simulink model "hpt_v2_topology2_paper"  (R2025a)
settings: Solver=ode23tb  StartTime=0.0  StopTime=0.2  RelTol=1e-3
model workspace (MAT data in the model file):
  hpt_chopper_threshold = 850
  hpt_conventional_energy_scale = 1
  hpt_conventional_energy_scale_sag = 1
  hpt_conventional_energy_scale_swell = 1
  hpt_conventional_recovery_hold_s = 0
  hpt_conventional_recovery_reg_gain = 0
  hpt_conventional_recovery_reg_max = 0
  hpt_conventional_reg_scale = 1
  hpt_conventional_reg_scale_sag = 1
  hpt_conventional_reg_scale_swell = 1
  hpt_ctrl_Ts = 2e-05
  hpt_energy_bridge_polarity = -1
  hpt_energy_control_sign = -1
  hpt_energy_i_ki = 100
  hpt_energy_i_kp = 0.5
  hpt_energy_id_max = 20
  hpt_energy_vff_gain = 1.06
  hpt_grid_f0 = 50
  hpt_inj_phase_offset = -1.05
  hpt_m_energy = 0
  hpt_m_energy_max = 0.95
  hpt_m_reg = 0.1
  hpt_m_reg_max = 0.8
  hpt_pll_ki = 2500
  hpt_pll_kp = 80
  hpt_pwm_fs = 2000
  hpt_rchop = 5.33333333333
  hpt_reg_openloop_amp = 0
  hpt_reg_openloop_phase = 0
  hpt_reg_polarity = 1
  hpt_s2_resistance = 0.001
  hpt_sac_actor_filter_tau = 0.001
  hpt_sac_actor_select_mode = 0
  hpt_sac_dynamic_reg_limit = 0.6
  hpt_sac_enable = 0
  hpt_sac_energy_enable = 0
  hpt_sac_energy_max = 0.95
  hpt_sac_fault_time_norm_s = 0.5
  hpt_sac_fixed_energy_d = 0
  hpt_sac_fixed_energy_q = 0
  hpt_sac_fixed_reg_d = 0
  hpt_sac_fixed_reg_q = 0
  hpt_sac_grid_vref_phase = 5773.5026919
  hpt_sac_gridnorm_startup_s = 0.03
  hpt_sac_guard_enable = 0
  hpt_sac_i_base_peak = 816.496580928
  hpt_sac_phase_fault_clear_s = 0
  hpt_sac_phase_fault_start_s = 0
  hpt_sac_phase_override_enable = 0
  hpt_sac_phase_recovery_end_s = 0
  hpt_sac_policy_mode = 0
  hpt_sac_recovery_time_norm_s = 0.5
  hpt_sac_reg_d_gain = 1
  hpt_sac_reg_max = 0.8
  hpt_sac_reg_polarity = 1
  hpt_sac_reg_q_gain = 1
  hpt_sac_topology_id = 2
  hpt_sac_vdc_ref = 800
  hpt_sac_vref_phase = 230
  hpt_swell_gain_scale = 1
  hpt_swell_m_reg_max = 0.5
  hpt_swell_phase_offset = -0.5
  hpt_traj_action = [0  0  0  0; 0  0  0  0; 0  0  0  0; 0  0  0  0; 0  0  0  0; 0  0  0  0; 0  0  0  0; 0  0  0  0; 0  0  0  0; 0  0  0  0; 0  0  0  0; 0  0  0  0; 0  0  0  0; 0  0  0  0; 0  0  0  0; 0  0  0  0; 0  0  0  0; 0  0  0  0; 0  0  0  0; 0  0  0  0; 0  0  0  0; 0  0  0  0; 0  0  0  0; 0  0  0  0; 0  0  0  0; 0  0  0  0; 0  0  0  0; 0  0  0  0; 0  0  0  0; 0  0  0  0; 0  0  0  0; 0  0  0  0; 0  0  0  0; 0  0  0  0; 0  0  0  0; 0  0  0  0; 0  0  0  0; 0  0  0  0; 0  0  0  0; 0  0  0  0; 0  0  0  0; 0  0  0  0; 0  0  0  0; 0  0  0  0; 0  0  0  0; 0  0  0  0; 0  0  0  0; 0  0  0  0; 0  0  0  0; 0  0  0  0; 0  0  0  0; 0  0  0  0; 0  0  0  0; 0  0  0  0; 0  0  0  0; 0  0  0  0; 0  0  0  0; 0  0  0  0; 0  0  0  0; 0  0  0  0; 0  0  0  0; 0  0  0  0; 0  0  0  0; 0  0  0  0; 0  0  0  0; 0  0  0  0; 0  0  0  0; 0  0  0  0; 0  0  0  0; 0  0  0  0; 0  0  0  0; 0  0  0  0; 0  0  0  0; 0  0  0  0; 0  0  0  0; 0  0  0  0; 0  0  0  0; 0  0  0  0; 0  0  0  0; 0  0  0  0; 0  0  0  0; 0  0  0  0; 0  0  0  0; 0  0  0  0; 0  0  0  0; 0  0  0  0; 0  0  0  0; 0  0  0  0; 0  0  0  0; 0  0  0  0; 0  0  0  0; 0  0  0  0; 0  0  0  0; 0  0  0  0; 0  0  0  0; 0  0  0  0; 0  0  0  0; 0  0  0  0; 0  0  0  0; 0  0  0  0; 0  0  0  0; 0  0  0  0; 0  0  0  0; 0  0  0  0; 0  0  0  0; 0  0  0  0; 0  0  0  0; 0  0  0  0; 0  0  0  0; 0  0  0  0; 0  0  0  0; 0  0  0  0; 0  0  0  0; 0  0  0  0; 0  0  0  0; 0  0  0  0; 0  0  0  0; 0  0  0  0; 0  0  0  0; 0  0  0  0; 0  0  0  0; 0  0  0  0; 0  0  0  0; 0  0  0  0; 0  0  0  0; 0  0  0  0]
  hpt_traj_t = [0; 0.002; 0.004; 0.006; 0.008; 0.01; 0.012; 0.014; 0.016; 0.018; 0.02; 0.022; 0.024; 0.026; 0.028; 0.03; 0.032; 0.034; 0.036; 0.038; 0.04; 0.042; 0.044; 0.046; 0.048; 0.05; 0.052; 0.054; 0.056; 0.058; 0.06; 0.062; 0.064; 0.066; 0.068; 0.07; 0.072; 0.074; 0.076; 0.078; 0.08; 0.082; 0.084; 0.086; 0.088; 0.09; 0.092; 0.094; 0.096; 0.098; 0.1; 0.102; 0.104; 0.106; 0.108; 0.11; 0.112; 0.114; 0.116; 0.118; 0.12; 0.122; 0.124; 0.126; 0.128; 0.13; 0.132; 0.134; 0.136; 0.138; 0.14; 0.142; 0.144; 0.146; 0.148; 0.15; 0.152; 0.154; 0.156; 0.158; 0.16; 0.162; 0.164; 0.166; 0.168; 0.17; 0.172; 0.174; 0.176; 0.178; 0.18; 0.182; 0.184; 0.186; 0.188; 0.19; 0.192; 0.194; 0.196; 0.198; 0.2; 0.202; 0.204; 0.206; 0.208; 0.21; 0.212; 0.214; 0.216; 0.218; 0.22; 0.222; 0.224; 0.226; 0.228; 0.23; 0.232; 0.234; 0.236; 0.238; 0.24; 0.242; 0.244; 0.246; 0.248; 0.25]
  hpt_vdc_ki = 0.2
  hpt_vdc_kp = 2
  hpt_vdc_ref = 800
  hpt_vref_lv = 207
  hpt_vreg_ki = 0
  hpt_vreg_kp = 20
libraries: spsSeriesRLCBranchLib x17, spsVoltageMeasurementLib x10, spsLinearTransformerLib x9, simulink x9, spsGroundLib x5, spsUniversalBridgeLib x4, spsThreePhaseVIMeasurementLib x3, spsCurrentMeasurementLib x3, spsIGBTLib x1, spsThreePhaseSourceLib x1, spsThreePhaseSeriesRLCLoadLib x1, spsThreePhaseSeriesRLCBranchLib x1
(part 1 of 2)
settings Model: Creator=m1391  LastModifiedBy=m1391

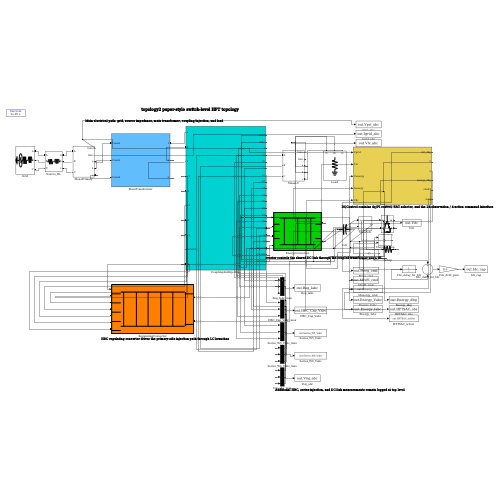
[thumbnail: Simulink's stored preview of the top-level diagram]
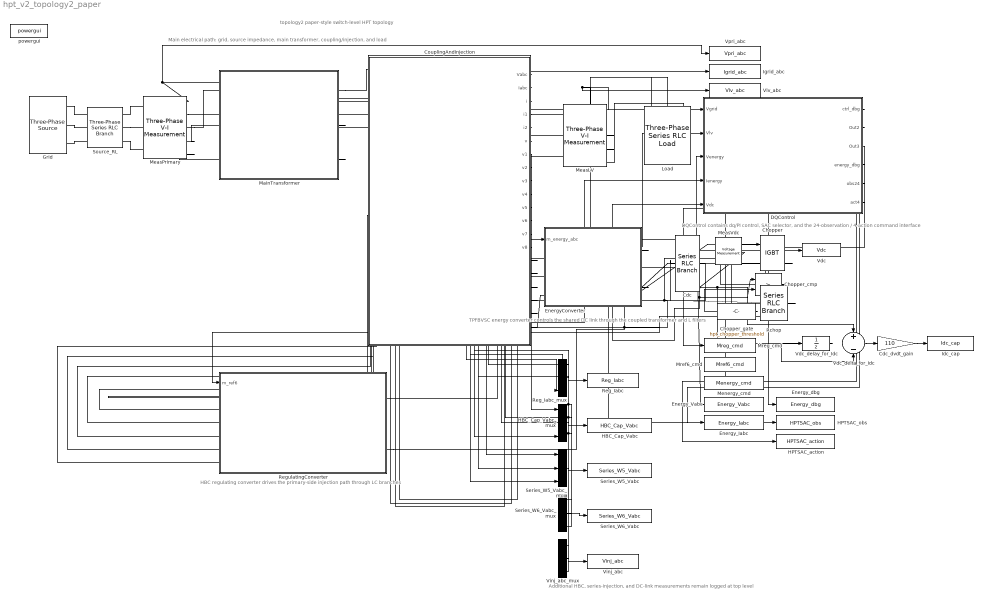
== system hpt_v2_topology2_paper ==
  note: topology2 paper-style switch-level HPT topology
  note: Main electrical path: grid, source impedance, main transformer, coupling/injection, and load
  note: HBC regulating converter drives the primary-side injection path through LC branches
  note: TPFBVSC energy converter controls the shared DC link through the coupled transformer and L filters
  note: DQControl contains dq/PI control, SAC selector, and the 24-observation / 4-action command interface
  note: Additional HBC, series-injection, and DC-link measurements remain logged at top level
  Cdc : spsSeriesRLCBranchLib/Series RLC Branch  LConnTagsString=__new0  RConnTagsString=__new0  BranchType=C  Resistance=1  Inductance=1e-3  SetiL0=off  InitialCurrent=0  Capacitance=0.0022  Setx0=on  InitialVoltage=800  Measurements=None
  Cdc_dvdt_gain : Gain  Gain=110
  Chopper : spsIGBTLib/IGBT  Ron=0.001  Lon=0  Vf=1  Tf=1e-6  Tt=2e-6  IC=0  Rs=1e5  Cs=inf  Measurements=on
  Chopper_cmp : RelationalOperator  Operator=>  OutDataTypeStr=boolean  RndMeth=Simplest  InputSameDT=off
  Chopper_gate : Constant  Value=hpt_chopper_threshold
  CouplingAndInjection : Subsystem
  DQControl : Subsystem
  EnergyConverter : Subsystem
      mask Display:
      | color('black');
      | plot([10 90 90 10 10],[10 10 90 90 10]);
      | plot([20 80],[78 78]); plot([20 80],[22 22]);
      | plot([28 28],[22 78]); plot([50 50],[22 78]); plot([72 72],[22 78]);
      | plot([10 20],[65 65]); plot([10 20],[50 50]); plot([10 20],[35 35]);
      | plot([80 90],[65 65]); plot([80 90],[35 35]);
  Energy_Iabc : ToWorkspace  VariableName=Energy_Iabc  SampleTime=2e-05
  Energy_Vabc : ToWorkspace  VariableName=Energy_Vabc  SampleTime=2e-05
  Energy_dbg : ToWorkspace  VariableName=Energy_dbg  SampleTime=2e-05
  Grid : spsThreePhaseSourceLib/Three-Phase Source  InternalConnection=Yg  VoltagePhases=off  Voltage=10000  PhaseAngle=0  Voltage_phases=[25e3 25e3 25e3]/sqrt(3)  PhaseAngles_phases=[0 -120 +120]  Frequency=50  NonIdealSource=on  SpecifyImpedance=off  Resistance=0.8929  Inductance=16.58e-3  ShortCircuitLevel=100e6  BaseVoltage=25e3  XRratio=7  BusType=swing  Pref=10e3  Qref=0  Prefabc=[10e3, 10e3, 10e3]  Qrefabc=[0, 0, 0]  Qmin=-inf  Qmax=inf
  HBC_Cap_Vabc : ToWorkspace  VariableName=HBC_Cap_Vabc  SampleTime=2e-05
  HBC_Cap_Vabc_mux : Mux  Inputs=3
  HPTSAC_action : ToWorkspace  VariableName=HPTSAC_action  SampleTime=2e-05
  HPTSAC_obs : ToWorkspace  VariableName=HPTSAC_obs  SampleTime=2e-05
  Idc_cap : ToWorkspace  VariableName=Idc_cap  SampleTime=2e-05
  Igrid_abc : ToWorkspace  VariableName=Igrid_abc  SampleTime=2e-05
  Load : spsThreePhaseSeriesRLCLoadLib/Three-Phase Series RLC Load  LConnTagsString=A|B|C  Configuration=Y (grounded)  NominalVoltage=400  Vabc=[1e3 1e3 1e3]  Vabcp=[1e3 1e3 1e3]  NominalFrequency=50  UnbalancedPower=off  ActivePower=400000  InductivePower=0  CapacitivePower=0  Pabc=[10e3 9e3 11e3]  QLabc=[100 90 110]  QCabc=[100 90 110]  Pabcp=[10e3 9e3 11e3]  QLabcp=[100 90 110]  QCabcp=[100 90 110]  Measurements=None  LoadType=constant Z
  MainTransformer : Subsystem
  MeasLV : spsThreePhaseVIMeasurementLib/Three-Phase V-I Measurement  VoltageMeasurement=phase-to-ground  SetLabelV=off  LabelV=Vabc  Vpu=off  VpuLL=off  CurrentMeasurement=yes  SetLabelI=off  LabelI=Iabc  Ipu=off  Pbase=100e6  Vbase=500e3  OutputType=Complex  PhasorSimulation=off  PSBequivalent=0
  MeasPrimary : spsThreePhaseVIMeasurementLib/Three-Phase V-I Measurement  VoltageMeasurement=phase-to-ground  SetLabelV=off  LabelV=Vabc  Vpu=off  VpuLL=off  CurrentMeasurement=yes  SetLabelI=off  LabelI=Iabc  Ipu=off  Pbase=100e6  Vbase=500e3  OutputType=Complex  PhasorSimulation=off  PSBequivalent=0
  MeasVdc : spsVoltageMeasurementLib/Voltage Measurement  PhasorSimulation=off  OutputType=Complex  PSBequivalent=0
  Menergy_cmd : ToWorkspace  VariableName=Menergy_cmd  SampleTime=2e-05
  Mref6_cmd : ToWorkspace  VariableName=Mref6_cmd  SampleTime=2e-05
  Mreg_cmd : ToWorkspace  VariableName=Mreg_cmd  SampleTime=2e-05
  Rchop : spsSeriesRLCBranchLib/Series RLC Branch  LConnTagsString=__new0  RConnTagsString=__new0  BranchType=R  Resistance=hpt_rchop  Inductance=1e-3  SetiL0=off  InitialCurrent=0  Capacitance=1e-6  Setx0=off  InitialVoltage=0  Measurements=None
  Reg_Iabc : ToWorkspace  VariableName=Reg_Iabc  SampleTime=2e-05
  Reg_Iabc_mux : Mux  Inputs=3
  RegulatingConverter : Subsystem
      mask Display:
      | color('black');
      | plot([5 95 95 5 5],[10 10 90 90 10]);
      | plot([15 85],[78 78]); plot([15 85],[22 22]);
      | plot([18 18],[22 78]); plot([32 32],[22 78]);
      | plot([45 45],[22 78]); plot([59 59],[22 78]);
      | plot([72 72],[22 78]); plot([86 86],[22 78]);
      | plot([5 15],[75 75]); plot([5 15],[60 60]); plot([5 15],[45 45]);
      | plot([5 15],[30 30]); plot([5 15],[15 15]); plot([5 15],[10 10]);
      | plot([85 95],[75 75]); plot([85 95],[25 25]);
  Series_W5_Vabc : ToWorkspace  VariableName=Series_W5_Vabc  SampleTime=2e-05
  Series_W5_Vabc_mux : Mux  Inputs=3
  Series_W6_Vabc : ToWorkspace  VariableName=Series_W6_Vabc  SampleTime=2e-05
  Series_W6_Vabc_mux : Mux  Inputs=3
  Source_RL : spsThreePhaseSeriesRLCBranchLib/Three-Phase Series RLC Branch  LConnTagsString=A|B|C  RConnTagsString=A|B|C  BranchType=RL  Resistance=11.7851  Inductance=0.26259  Capacitance=1e-6  Measurements=None
  Vdc : ToWorkspace  VariableName=Vdc  SampleTime=2e-05
  Vdc_delay_for_Idc : UnitDelay  InitialCondition=800  SampleTime=2e-05  HasFrameUpgradeWarning=on
  Vdc_delta_for_Idc : Sum  Inputs=+-
  Vinj_abc : ToWorkspace  VariableName=Vinj_abc  SampleTime=2e-05
  Vinj_abc_mux : Mux  Inputs=3
  Vlv_abc : ToWorkspace  VariableName=Vlv_abc  SampleTime=2e-05
  Vpri_abc : ToWorkspace  VariableName=Vpri_abc  SampleTime=2e-05
  powergui : spspowerguiLib/powergui  Priority=1  SimulationMode=Discrete  SampleTime=2e-05  frequency=60  Iterations=50  frequencyindice=60  Pbase=100e6  ErrMax=1e-4  UnitsV=kV  UnitsW=MW  buscounter=0  FunctionMessages=off  echomessages=off  EnableUseOfTLC=off  CurrentSourceSwitches=off  DisableSnubberDevices=off  DisableRonSwitches=off  DisableVfSwitches=off  DisplayEquations=off  AutomaticDiscreteSolvers=off  SolverType=Tustin/Backward Euler (TBE)  Interpol=off  ExternalGateDelay=off  methode=off  Ts=100  x0status=blocks  SPID=on  SwTol=0  HookPort=off  NonlinearTolerance=1e-4  nMaxIteration=100  ContinueOnMaxIteration=off  RestoreLinks=warning  ResistiveCurrentMeasurement=off  Frange=[0:2:500]  Ylog=off  Xlog=on  ShowGrid=off  save=off  variable=ZData  structure=0  ZoomFFT=off  StartTime=0.0  cycles=1  DisplayStyle=1  fundamental=60  FreqAxis=off  MaxFrequency=1000  frequencyindicesteady=1  RmsSteady=1  display=off
  wires:
  MeasVdc/1 -> DQControl/5(Vdc), Chopper_cmp/1, Vdc_delay_for_Idc/1, Vdc_delta_for_Idc/1, Vdc/1
  Chopper_gate/1 -> Chopper_cmp/2
  Chopper_cmp/1 -> Chopper/1
  MeasPrimary/1 -> DQControl/1(Vgrid), Vpri_abc/1
  MeasPrimary/2 -> Igrid_abc/1
  MeasLV/1 -> DQControl/2(Vlv), Vlv_abc/1
  Vdc_delay_for_Idc/1 -> Vdc_delta_for_Idc/2
  Vdc_delta_for_Idc/1 -> Cdc_dvdt_gain/1
  Cdc_dvdt_gain/1 -> Idc_cap/1
  Reg_Iabc_mux/1 -> Reg_Iabc/1
  HBC_Cap_Vabc_mux/1 -> HBC_Cap_Vabc/1
  Series_W5_Vabc_mux/1 -> Series_W5_Vabc/1
  Series_W6_Vabc_mux/1 -> Series_W6_Vabc/1
  Vinj_abc_mux/1 -> Vinj_abc/1
  CouplingAndInjection/8(v2) -> Series_W6_Vabc_mux/2, Vinj_abc_mux/2
  CouplingAndInjection/6(v) -> Series_W6_Vabc_mux/1, Vinj_abc_mux/1
  CouplingAndInjection/10(v4) -> Series_W6_Vabc_mux/3, Vinj_abc_mux/3
  CouplingAndInjection/2(Iabc) -> DQControl/4(Ienergy), Energy_Iabc/1
  CouplingAndInjection/1(Vabc) -> DQControl/3(Venergy), Energy_Vabc/1
  CouplingAndInjection/3(i) -> Reg_Iabc_mux/1
  CouplingAndInjection/4(i1) -> Reg_Iabc_mux/2
  CouplingAndInjection/5(i2) -> Reg_Iabc_mux/3
  CouplingAndInjection/7(v1) -> HBC_Cap_Vabc_mux/1
  CouplingAndInjection/9(v3) -> HBC_Cap_Vabc_mux/2
  CouplingAndInjection/11(v5) -> HBC_Cap_Vabc_mux/3
  CouplingAndInjection/12(v6) -> Series_W5_Vabc_mux/1
  CouplingAndInjection/13(v7) -> Series_W5_Vabc_mux/2
  CouplingAndInjection/14(v8) -> Series_W5_Vabc_mux/3
  DQControl/2(Out2) -> RegulatingConverter/1(m_ref6), Mref6_cmd/1
  DQControl/3(Out3) -> Menergy_cmd/1, EnergyConverter/1(m_energy_abc)
  DQControl/1(ctrl_dbg) -> Mreg_cmd/1
  DQControl/4(energy_dbg) -> Energy_dbg/1
  DQControl/5(obs24) -> HPTSAC_obs/1
  DQControl/6(act4) -> HPTSAC_action/1
  connections:
  Grid/RConn1 -- Source_RL/LConn1
  Source_RL/RConn1 -- MeasPrimary/LConn1
  MeasLV/RConn1 -- Load/LConn1
  Grid/RConn2 -- Source_RL/LConn2
  Source_RL/RConn2 -- MeasPrimary/LConn2
  MeasLV/RConn2 -- Load/LConn2
  Grid/RConn3 -- Source_RL/LConn3
  Source_RL/RConn3 -- MeasPrimary/LConn3
  MeasLV/RConn3 -- Load/LConn3
  EnergyConverter/RConn1 -- Cdc/LConn1 -- MeasVdc/LConn1 -- Chopper/LConn1 -- RegulatingConverter/RConn1
  EnergyConverter/RConn2 -- Cdc/RConn1 -- Rchop/RConn1 -- MeasVdc/LConn2 -- RegulatingConverter/RConn2
  Chopper/RConn1 -- Rchop/LConn1
  MeasPrimary/RConn1 -- MainTransformer/LConn1
  MeasPrimary/RConn2 -- MainTransformer/LConn2
  MeasPrimary/RConn3 -- MainTransformer/LConn3
  CouplingAndInjection/RConn1 -- MeasLV/LConn1
  CouplingAndInjection/RConn2 -- MeasLV/LConn2
  CouplingAndInjection/RConn3 -- MeasLV/LConn3
  MainTransformer/RConn1 -- CouplingAndInjection/LConn1
  MainTransformer/RConn2 -- CouplingAndInjection/LConn2
  MainTransformer/RConn3 -- CouplingAndInjection/LConn3
  CouplingAndInjection/RConn4 -- EnergyConverter/LConn1
  CouplingAndInjection/RConn5 -- EnergyConverter/LConn2
  CouplingAndInjection/RConn6 -- EnergyConverter/LConn3
  RegulatingConverter/LConn1 -- CouplingAndInjection/LConn4
  RegulatingConverter/LConn2 -- CouplingAndInjection/LConn5
  RegulatingConverter/LConn3 -- CouplingAndInjection/LConn6
  RegulatingConverter/LConn4 -- CouplingAndInjection/LConn7
  RegulatingConverter/LConn5 -- CouplingAndInjection/LConn8
  RegulatingConverter/LConn6 -- CouplingAndInjection/LConn10

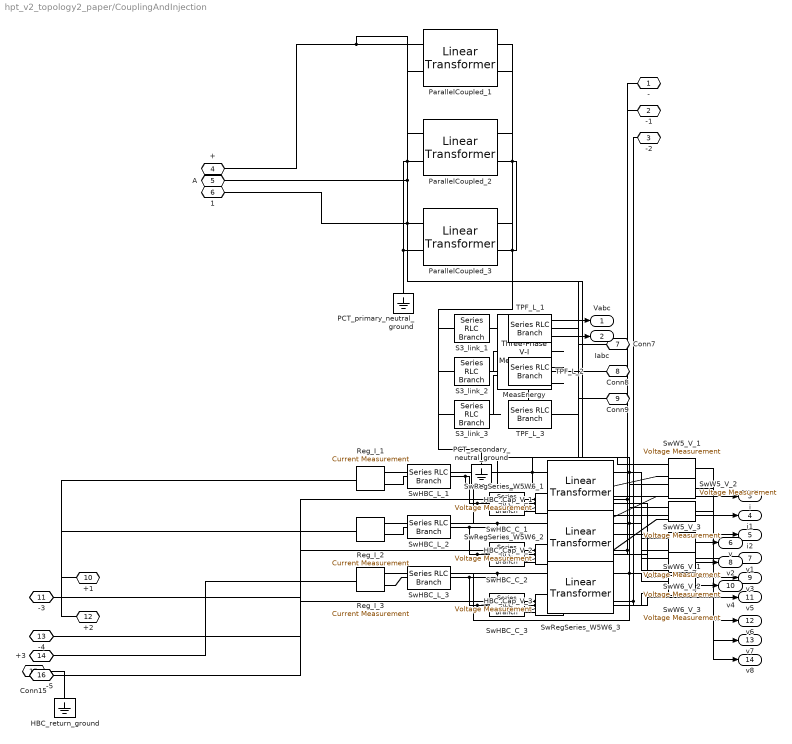
== system hpt_v2_topology2_paper/CouplingAndInjection ==
  HBC_Cap_V_1 : spsVoltageMeasurementLib/Voltage Measurement  PhasorSimulation=off  OutputType=Complex  PSBequivalent=0
  HBC_Cap_V_2 : spsVoltageMeasurementLib/Voltage Measurement  PhasorSimulation=off  OutputType=Complex  PSBequivalent=0
  HBC_Cap_V_3 : spsVoltageMeasurementLib/Voltage Measurement  PhasorSimulation=off  OutputType=Complex  PSBequivalent=0
  HBC_return_ground : spsGroundLib/Ground  LConnTagsString=a
  MeasEnergy : spsThreePhaseVIMeasurementLib/Three-Phase V-I Measurement  VoltageMeasurement=phase-to-ground  SetLabelV=off  LabelV=Vabc  Vpu=off  VpuLL=off  CurrentMeasurement=yes  SetLabelI=off  LabelI=Iabc  Ipu=off  Pbase=100e6  Vbase=500e3  OutputType=Complex  PhasorSimulation=off  PSBequivalent=0
  PCT_primary_neutral_ground : spsGroundLib/Ground  LConnTagsString=a
  PCT_secondary_neutral_ground : spsGroundLib/Ground  LConnTagsString=a
  ParallelCoupled_1 : spsLinearTransformerLib/Linear Transformer  UNITS=pu  NominalPower=[40000,50]  winding1=[230.9401,0.004,0.02]  winding2=[230.9401,0.004,0.02]  ThreeWindings=off  winding3=[ 315e3 0.002 0.08 ]  RmLm=[ 500 500 ]  Measurements=None  DataType=off
  ParallelCoupled_2 : spsLinearTransformerLib/Linear Transformer  UNITS=pu  NominalPower=[40000,50]  winding1=[230.9401,0.004,0.02]  winding2=[230.9401,0.004,0.02]  ThreeWindings=off  winding3=[ 315e3 0.002 0.08 ]  RmLm=[ 500 500 ]  Measurements=None  DataType=off
  ParallelCoupled_3 : spsLinearTransformerLib/Linear Transformer  UNITS=pu  NominalPower=[40000,50]  winding1=[230.9401,0.004,0.02]  winding2=[230.9401,0.004,0.02]  ThreeWindings=off  winding3=[ 315e3 0.002 0.08 ]  RmLm=[ 500 500 ]  Measurements=None  DataType=off
  Reg_I_1 : spsCurrentMeasurementLib/Current Measurement  PhasorSimulation=off  OutputType=Complex  PSBequivalent=0
  Reg_I_2 : spsCurrentMeasurementLib/Current Measurement  PhasorSimulation=off  OutputType=Complex  PSBequivalent=0
  Reg_I_3 : spsCurrentMeasurementLib/Current Measurement  PhasorSimulation=off  OutputType=Complex  PSBequivalent=0
  S3_link_1 : spsSeriesRLCBranchLib/Series RLC Branch  LConnTagsString=__new0  RConnTagsString=__new0  BranchType=R  Resistance=1e-3  Inductance=1e-3  SetiL0=off  InitialCurrent=0  Capacitance=1e-6  Setx0=off  InitialVoltage=0  Measurements=None
  S3_link_2 : spsSeriesRLCBranchLib/Series RLC Branch  LConnTagsString=__new0  RConnTagsString=__new0  BranchType=R  Resistance=1e-3  Inductance=1e-3  SetiL0=off  InitialCurrent=0  Capacitance=1e-6  Setx0=off  InitialVoltage=0  Measurements=None
  S3_link_3 : spsSeriesRLCBranchLib/Series RLC Branch  LConnTagsString=__new0  RConnTagsString=__new0  BranchType=R  Resistance=1e-3  Inductance=1e-3  SetiL0=off  InitialCurrent=0  Capacitance=1e-6  Setx0=off  InitialVoltage=0  Measurements=None
  SwHBC_C_1 : spsSeriesRLCBranchLib/Series RLC Branch  LConnTagsString=__new0  RConnTagsString=__new0  BranchType=C  Resistance=1  Inductance=1e-3  SetiL0=off  InitialCurrent=0  Capacitance=2e-05  Setx0=off  InitialVoltage=0  Measurements=None
  SwHBC_C_2 : spsSeriesRLCBranchLib/Series RLC Branch  LConnTagsString=__new0  RConnTagsString=__new0  BranchType=C  Resistance=1  Inductance=1e-3  SetiL0=off  InitialCurrent=0  Capacitance=2e-05  Setx0=off  InitialVoltage=0  Measurements=None
  SwHBC_C_3 : spsSeriesRLCBranchLib/Series RLC Branch  LConnTagsString=__new0  RConnTagsString=__new0  BranchType=C  Resistance=1  Inductance=1e-3  SetiL0=off  InitialCurrent=0  Capacitance=2e-05  Setx0=off  InitialVoltage=0  Measurements=None
  SwHBC_L_1 : spsSeriesRLCBranchLib/Series RLC Branch  LConnTagsString=__new0  RConnTagsString=__new0  BranchType=RL  Resistance=0.03  Inductance=0.002  SetiL0=off  InitialCurrent=0  Capacitance=1e-6  Setx0=off  InitialVoltage=0  Measurements=None
  SwHBC_L_2 : spsSeriesRLCBranchLib/Series RLC Branch  LConnTagsString=__new0  RConnTagsString=__new0  BranchType=RL  Resistance=0.03  Inductance=0.002  SetiL0=off  InitialCurrent=0  Capacitance=1e-6  Setx0=off  InitialVoltage=0  Measurements=None
  SwHBC_L_3 : spsSeriesRLCBranchLib/Series RLC Branch  LConnTagsString=__new0  RConnTagsString=__new0  BranchType=RL  Resistance=0.03  Inductance=0.002  SetiL0=off  InitialCurrent=0  Capacitance=1e-6  Setx0=off  InitialVoltage=0  Measurements=None
  SwRegSeries_W5W6_1 : spsLinearTransformerLib/Linear Transformer  UNITS=pu  NominalPower=[30000,50]  winding1=[400,0.002,0.03]  winding2=[100,0.002,0.03]  ThreeWindings=off  winding3=[ 315e3 0.002 0.08 ]  RmLm=[ 500 500 ]  Measurements=None  DataType=off
  SwRegSeries_W5W6_2 : spsLinearTransformerLib/Linear Transformer  UNITS=pu  NominalPower=[30000,50]  winding1=[400,0.002,0.03]  winding2=[100,0.002,0.03]  ThreeWindings=off  winding3=[ 315e3 0.002 0.08 ]  RmLm=[ 500 500 ]  Measurements=None  DataType=off
  SwRegSeries_W5W6_3 : spsLinearTransformerLib/Linear Transformer  UNITS=pu  NominalPower=[30000,50]  winding1=[400,0.002,0.03]  winding2=[100,0.002,0.03]  ThreeWindings=off  winding3=[ 315e3 0.002 0.08 ]  RmLm=[ 500 500 ]  Measurements=None  DataType=off
  SwW5_V_1 : spsVoltageMeasurementLib/Voltage Measurement  PhasorSimulation=off  OutputType=Complex  PSBequivalent=0
  SwW5_V_2 : spsVoltageMeasurementLib/Voltage Measurement  PhasorSimulation=off  OutputType=Complex  PSBequivalent=0
  SwW5_V_3 : spsVoltageMeasurementLib/Voltage Measurement  PhasorSimulation=off  OutputType=Complex  PSBequivalent=0
  SwW6_V_1 : spsVoltageMeasurementLib/Voltage Measurement  PhasorSimulation=off  OutputType=Complex  PSBequivalent=0
  SwW6_V_2 : spsVoltageMeasurementLib/Voltage Measurement  PhasorSimulation=off  OutputType=Complex  PSBequivalent=0
  SwW6_V_3 : spsVoltageMeasurementLib/Voltage Measurement  PhasorSimulation=off  OutputType=Complex  PSBequivalent=0
  TPF_L_1 : spsSeriesRLCBranchLib/Series RLC Branch  LConnTagsString=__new0  RConnTagsString=__new0  BranchType=L  Resistance=1  Inductance=0.0015  SetiL0=off  InitialCurrent=0  Capacitance=1e-6  Setx0=off  InitialVoltage=0  Measurements=None
  TPF_L_2 : spsSeriesRLCBranchLib/Series RLC Branch  LConnTagsString=__new0  RConnTagsString=__new0  BranchType=L  Resistance=1  Inductance=0.0015  SetiL0=off  InitialCurrent=0  Capacitance=1e-6  Setx0=off  InitialVoltage=0  Measurements=None
  TPF_L_3 : spsSeriesRLCBranchLib/Series RLC Branch  LConnTagsString=__new0  RConnTagsString=__new0  BranchType=L  Resistance=1  Inductance=0.0015  SetiL0=off  InitialCurrent=0  Capacitance=1e-6  Setx0=off  InitialVoltage=0  Measurements=None
  - : PMIOPort  Side=Right
  -1 : PMIOPort  Port=2  Side=Right
  -2 : PMIOPort  Port=3  Side=Right
  + : PMIOPort  Port=4  Side=Left
  A : PMIOPort  Port=5  Side=Left
  1 : PMIOPort  Port=6  Side=Left
  Conn7 : PMIOPort  Port=7  Side=Right
  Conn8 : PMIOPort  Port=8  Side=Right
  Conn9 : PMIOPort  Port=9  Side=Right
  +1 : PMIOPort  Port=10  Side=Left
  -3 : PMIOPort  Port=11  Side=Left
  +2 : PMIOPort  Port=12  Side=Left
  -4 : PMIOPort  Port=13  Side=Left
  +3 : PMIOPort  Port=14  Side=Left
  Conn15 : PMIOPort  Port=15  Side=Left
  -5 : PMIOPort  Port=16  Side=Left
  Vabc : Outport
  Iabc : Outport  Port=2
  i : Outport  Port=3
  i1 : Outport  Port=4
  i2 : Outport  Port=5
  v : Outport  Port=6
  v1 : Outport  Port=7
  v2 : Outport  Port=8
  v3 : Outport  Port=9
  v4 : Outport  Port=10
  v5 : Outport  Port=11
  v6 : Outport  Port=12
  v7 : Outport  Port=13
  v8 : Outport  Port=14
  wires:
  Reg_I_2/1 -> i1/1
  Reg_I_1/1 -> i/1
  MeasEnergy/2 -> Iabc/1
  SwW5_V_3/1 -> v8/1
  Reg_I_3/1 -> i2/1
  HBC_Cap_V_3/1 -> v5/1
  SwW6_V_1/1 -> v/1
  SwW6_V_3/1 -> v4/1
  SwW5_V_1/1 -> v6/1
  SwW6_V_2/1 -> v2/1
  HBC_Cap_V_1/1 -> v1/1
  HBC_Cap_V_2/1 -> v3/1
  SwW5_V_2/1 -> v7/1
  MeasEnergy/1 -> Vabc/1
  connections:
  SwRegSeries_W5W6_3/RConn2 -- SwW6_V_3/LConn2 -- -2/RConn1
  ParallelCoupled_2/RConn1 -- S3_link_2/LConn1
  SwHBC_C_2/RConn1 -- HBC_Cap_V_2/LConn2 -- -4/RConn1 -- SwRegSeries_W5W6_2/LConn2 -- SwW5_V_2/LConn2
  ParallelCoupled_1/LConn1 -- +/RConn1 -- SwRegSeries_W5W6_1/RConn1 -- SwW6_V_1/LConn1
  SwRegSeries_W5W6_2/RConn2 -- SwW6_V_2/LConn2 -- -1/RConn1
  SwHBC_L_3/RConn1 -- SwHBC_C_3/LConn1 -- HBC_Cap_V_3/LConn1 -- SwRegSeries_W5W6_3/LConn1 -- SwW5_V_3/LConn1
  ParallelCoupled_1/RConn2 -- ParallelCoupled_2/RConn2 -- ParallelCoupled_3/RConn2 -- PCT_secondary_neutral_ground/LConn1
  SwHBC_C_3/RConn1 -- HBC_Cap_V_3/LConn2 -- -5/RConn1 -- SwRegSeries_W5W6_3/LConn2 -- SwW5_V_3/LConn2
  SwRegSeries_W5W6_1/RConn2 -- SwW6_V_1/LConn2 -- -/RConn1
  ParallelCoupled_3/LConn1 -- 1/RConn1 -- SwRegSeries_W5W6_3/RConn1 -- SwW6_V_3/LConn1
  +3/RConn1 -- Reg_I_3/LConn1
  MeasEnergy/RConn2 -- TPF_L_2/LConn1
  S3_link_1/RConn1 -- MeasEnergy/LConn1
  SwHBC_C_1/RConn1 -- HBC_Cap_V_1/LConn2 -- -3/RConn1 -- SwRegSeries_W5W6_1/LConn2 -- SwW5_V_1/LConn2
  A/RConn1 -- ParallelCoupled_2/LConn1 -- SwRegSeries_W5W6_2/RConn1 -- SwW6_V_2/LConn1
  ParallelCoupled_3/RConn1 -- S3_link_3/LConn1
  MeasEnergy/RConn1 -- TPF_L_1/LConn1
  Reg_I_1/RConn1 -- SwHBC_L_1/LConn1
  Reg_I_3/RConn1 -- SwHBC_L_3/LConn1
  SwHBC_L_2/RConn1 -- SwHBC_C_2/LConn1 -- HBC_Cap_V_2/LConn1 -- SwRegSeries_W5W6_2/LConn1 -- SwW5_V_2/LConn1
  MeasEnergy/RConn3 -- TPF_L_3/LConn1
  ParallelCoupled_1/RConn1 -- S3_link_1/LConn1
  ParallelCoupled_1/LConn2 -- ParallelCoupled_2/LConn2 -- ParallelCoupled_3/LConn2 -- PCT_primary_neutral_ground/LConn1
  S3_link_2/RConn1 -- MeasEnergy/LConn2
  SwHBC_L_1/RConn1 -- SwHBC_C_1/LConn1 -- HBC_Cap_V_1/LConn1 -- SwRegSeries_W5W6_1/LConn1 -- SwW5_V_1/LConn1
  HBC_return_ground/LConn1 -- Conn15/RConn1
  S3_link_3/RConn1 -- MeasEnergy/LConn3
  +1/RConn1 -- Reg_I_1/LConn1
  Reg_I_2/RConn1 -- SwHBC_L_2/LConn1
  TPF_L_3/RConn1 -- Conn9/RConn1
  TPF_L_2/RConn1 -- Conn8/RConn1
  TPF_L_1/RConn1 -- Conn7/RConn1
  +2/RConn1 -- Reg_I_2/LConn1

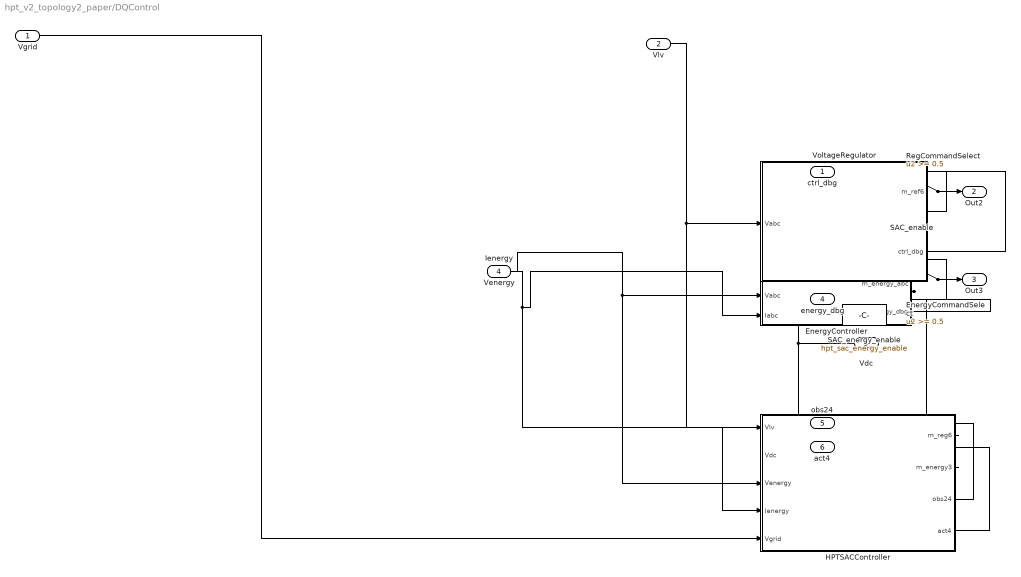
== system hpt_v2_topology2_paper/DQControl ==
  Vgrid : Inport
  Vlv : Inport  Port=2
  Venergy : Inport  Port=3
  Ienergy : Inport  Port=4
  Vdc : Inport  Port=5
  EnergyCommandSelect : Switch  Threshold=0.5  SaturateOnIntegerOverflow=off  InputSameDT=off
  EnergyController : Subsystem
  HPTSACController : Subsystem
  RegCommandSelect : Switch  Threshold=0.5  SaturateOnIntegerOverflow=off  InputSameDT=off
  SAC_enable : Constant  Value=hpt_sac_enable
  SAC_energy_enable : Constant  Value=hpt_sac_energy_enable
  VoltageRegulator : Subsystem
  ctrl_dbg : Outport
  Out2 : Outport  Port=2
  Out3 : Outport  Port=3
  energy_dbg : Outport  Port=4
  obs24 : Outport  Port=5
  act4 : Outport  Port=6
  wires:
  Venergy/1 -> EnergyController/2(Vabc), HPTSACController/3(Venergy)
  Ienergy/1 -> EnergyController/3(Iabc), HPTSACController/4(Ienergy)
  Vgrid/1 -> HPTSACController/5(Vgrid)
  HPTSACController/1(m_reg6) -> RegCommandSelect/1
  SAC_energy_enable/1 -> EnergyCommandSelect/2
  SAC_enable/1 -> RegCommandSelect/2
  HPTSACController/3(obs24) -> obs24/1
  Vdc/1 -> HPTSACController/2(Vdc), EnergyController/1(Vdc)
  VoltageRegulator/1(m_ref6) -> RegCommandSelect/3
  Vlv/1 -> VoltageRegulator/1(Vabc), HPTSACController/1(Vlv)
  HPTSACController/2(m_energy3) -> EnergyCommandSelect/1
  EnergyController/1(m_energy_abc) -> EnergyCommandSelect/3
  VoltageRegulator/2(ctrl_dbg) -> ctrl_dbg/1
  RegCommandSelect/1 -> Out2/1
  HPTSACController/4(act4) -> act4/1
  EnergyCommandSelect/1 -> Out3/1
  EnergyController/2(energy_dbg) -> energy_dbg/1

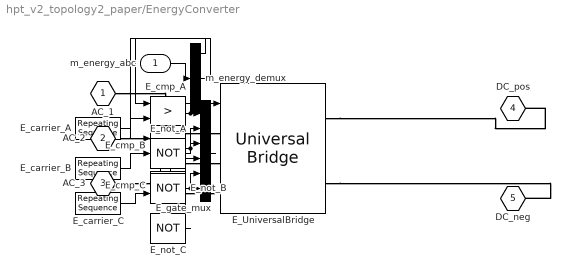
== system hpt_v2_topology2_paper/EnergyConverter ==
  m_energy_abc : Inport
  E_UniversalBridge : spsUniversalBridgeLib/Universal Bridge  Arms=3  SnubberResistance=1e5  SnubberCapacitance=inf  Device=IGBT / Diodes  Ron=1e-3  Lon=0  ForwardVoltages=[0.8 0.8]  ForwardVoltage=0  GTOparameters=[ 10e-6 , 20e-6 ]  IGBTparameters=[ 1e-6 , 2e-6 ]  Measurements=None  Measurements_2=None  converterType=Rectifier
  E_carrier_A : simulink/Sources/Repeating Sequence  rep_seq_t=[0 0.5/hpt_pwm_fs 1/hpt_pwm_fs]  rep_seq_y=[-1 1 -1]
  E_carrier_B : simulink/Sources/Repeating Sequence  rep_seq_t=[0 0.5/hpt_pwm_fs 1/hpt_pwm_fs]  rep_seq_y=[-1 1 -1]
  E_carrier_C : simulink/Sources/Repeating Sequence  rep_seq_t=[0 0.5/hpt_pwm_fs 1/hpt_pwm_fs]  rep_seq_y=[-1 1 -1]
  E_cmp_A : RelationalOperator  Operator=>  OutDataTypeStr=boolean  RndMeth=Simplest  InputSameDT=off
  E_cmp_B : RelationalOperator  Operator=>  OutDataTypeStr=boolean  RndMeth=Simplest  InputSameDT=off
  E_cmp_C : RelationalOperator  Operator=>  OutDataTypeStr=boolean  RndMeth=Simplest  InputSameDT=off
  E_gate_mux : Mux  Inputs=6
  E_not_A : Logic  Operator=NOT  AllPortsSameDT=off  OutDataTypeStr=boolean
  E_not_B : Logic  Operator=NOT  AllPortsSameDT=off  OutDataTypeStr=boolean
  E_not_C : Logic  Operator=NOT  AllPortsSameDT=off  OutDataTypeStr=boolean
  m_energy_demux : Demux  Outputs=3
  AC_1 : PMIOPort  Side=Left
  AC_2 : PMIOPort  Port=2  Side=Left
  AC_3 : PMIOPort  Port=3  Side=Left
  DC_pos : PMIOPort  Port=4  Side=Right
  DC_neg : PMIOPort  Port=5  Side=Right
  wires:
  m_energy_abc/1 -> m_energy_demux/1
  m_energy_demux/1 -> E_cmp_A/1
  E_carrier_A/1 -> E_cmp_A/2
  E_cmp_A/1 -> E_gate_mux/1, E_not_A/1
  E_not_A/1 -> E_gate_mux/2
  m_energy_demux/2 -> E_cmp_B/1
  E_carrier_B/1 -> E_cmp_B/2
  E_cmp_B/1 -> E_gate_mux/3, E_not_B/1
  E_not_B/1 -> E_gate_mux/4
  m_energy_demux/3 -> E_cmp_C/1
  E_carrier_C/1 -> E_cmp_C/2
  E_cmp_C/1 -> E_gate_mux/5, E_not_C/1
  E_not_C/1 -> E_gate_mux/6
  E_gate_mux/1 -> E_UniversalBridge/1
  connections:
  AC_1/RConn1 -- E_UniversalBridge/LConn1
  AC_2/RConn1 -- E_UniversalBridge/LConn2
  AC_3/RConn1 -- E_UniversalBridge/LConn3
  E_UniversalBridge/RConn1 -- DC_pos/RConn1
  E_UniversalBridge/RConn2 -- DC_neg/RConn1

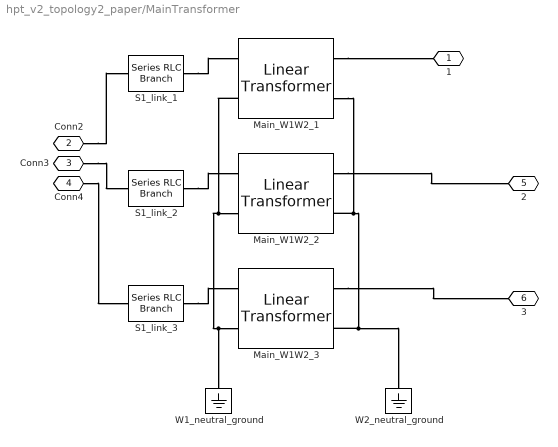
== system hpt_v2_topology2_paper/MainTransformer ==
  Main_W1W2_1 : spsLinearTransformerLib/Linear Transformer  UNITS=pu  NominalPower=[133333.3333,50]  winding1=[5773.5027,0.005,0.025]  winding2=[230.9401,0.005,0.025]  ThreeWindings=off  winding3=[ 315e3 0.002 0.08 ]  RmLm=[ 500 500 ]  Measurements=None  DataType=off
  Main_W1W2_2 : spsLinearTransformerLib/Linear Transformer  UNITS=pu  NominalPower=[133333.3333,50]  winding1=[5773.5027,0.005,0.025]  winding2=[230.9401,0.005,0.025]  ThreeWindings=off  winding3=[ 315e3 0.002 0.08 ]  RmLm=[ 500 500 ]  Measurements=None  DataType=off
  Main_W1W2_3 : spsLinearTransformerLib/Linear Transformer  UNITS=pu  NominalPower=[133333.3333,50]  winding1=[5773.5027,0.005,0.025]  winding2=[230.9401,0.005,0.025]  ThreeWindings=off  winding3=[ 315e3 0.002 0.08 ]  RmLm=[ 500 500 ]  Measurements=None  DataType=off
  S1_link_1 : spsSeriesRLCBranchLib/Series RLC Branch  LConnTagsString=__new0  RConnTagsString=__new0  BranchType=R  Resistance=1e-3  Inductance=1e-3  SetiL0=off  InitialCurrent=0  Capacitance=1e-6  Setx0=off  InitialVoltage=0  Measurements=None
  S1_link_2 : spsSeriesRLCBranchLib/Series RLC Branch  LConnTagsString=__new0  RConnTagsString=__new0  BranchType=R  Resistance=1e-3  Inductance=1e-3  SetiL0=off  InitialCurrent=0  Capacitance=1e-6  Setx0=off  InitialVoltage=0  Measurements=None
  S1_link_3 : spsSeriesRLCBranchLib/Series RLC Branch  LConnTagsString=__new0  RConnTagsString=__new0  BranchType=R  Resistance=1e-3  Inductance=1e-3  SetiL0=off  InitialCurrent=0  Capacitance=1e-6  Setx0=off  InitialVoltage=0  Measurements=None
  W1_neutral_ground : spsGroundLib/Ground  LConnTagsString=a
  W2_neutral_ground : spsGroundLib/Ground  LConnTagsString=a
  1 : PMIOPort  Side=Right
  Conn2 : PMIOPort  Port=2  Side=Left
  Conn3 : PMIOPort  Port=3  Side=Left
  Conn4 : PMIOPort  Port=4  Side=Left
  2 : PMIOPort  Port=5  Side=Right
  3 : PMIOPort  Port=6  Side=Right
  connections:
  S1_link_3/RConn1 -- Main_W1W2_3/LConn1
  Main_W1W2_1/LConn2 -- Main_W1W2_2/LConn2 -- Main_W1W2_3/LConn2 -- W1_neutral_ground/LConn1
  S1_link_1/RConn1 -- Main_W1W2_1/LConn1
  Main_W1W2_3/RConn1 -- 3/RConn1
  S1_link_2/RConn1 -- Main_W1W2_2/LConn1
  Main_W1W2_1/RConn2 -- Main_W1W2_2/RConn2 -- Main_W1W2_3/RConn2 -- W2_neutral_ground/LConn1
  Conn3/RConn1 -- S1_link_2/LConn1
  Main_W1W2_1/RConn1 -- 1/RConn1
  Conn2/RConn1 -- S1_link_1/LConn1
  Conn4/RConn1 -- S1_link_3/LConn1
  Main_W1W2_2/RConn1 -- 2/RConn1

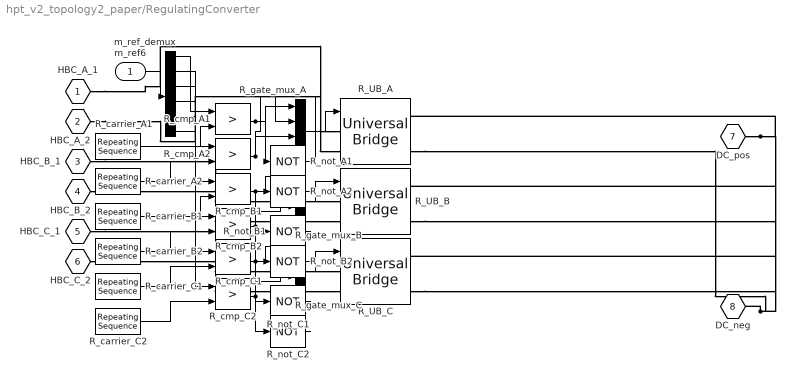
== system hpt_v2_topology2_paper/RegulatingConverter ==
  m_ref6 : Inport
  R_UB_A : spsUniversalBridgeLib/Universal Bridge  Arms=2  SnubberResistance=1e5  SnubberCapacitance=1e-9  Device=IGBT / Diodes  Ron=1e-3  Lon=0  ForwardVoltages="[  0  0  ]"  ForwardVoltage=0  GTOparameters=[ 10e-6 , 20e-6 ]  IGBTparameters=[ 1e-6 , 2e-6 ]  Measurements=None  Measurements_2=None  converterType=Rectifier
  R_UB_B : spsUniversalBridgeLib/Universal Bridge  Arms=2  SnubberResistance=1e5  SnubberCapacitance=1e-9  Device=IGBT / Diodes  Ron=1e-3  Lon=0  ForwardVoltages="[  0  0  ]"  ForwardVoltage=0  GTOparameters=[ 10e-6 , 20e-6 ]  IGBTparameters=[ 1e-6 , 2e-6 ]  Measurements=None  Measurements_2=None  converterType=Rectifier
  R_UB_C : spsUniversalBridgeLib/Universal Bridge  Arms=2  SnubberResistance=1e5  SnubberCapacitance=1e-9  Device=IGBT / Diodes  Ron=1e-3  Lon=0  ForwardVoltages="[  0  0  ]"  ForwardVoltage=0  GTOparameters=[ 10e-6 , 20e-6 ]  IGBTparameters=[ 1e-6 , 2e-6 ]  Measurements=None  Measurements_2=None  converterType=Rectifier
  R_carrier_A1 : simulink/Sources/Repeating Sequence  rep_seq_t=[0 0.5/hpt_pwm_fs 1/hpt_pwm_fs]  rep_seq_y=[-1 1 -1]
  R_carrier_A2 : simulink/Sources/Repeating Sequence  rep_seq_t=[0 0.5/hpt_pwm_fs 1/hpt_pwm_fs]  rep_seq_y=[-1 1 -1]
  R_carrier_B1 : simulink/Sources/Repeating Sequence  rep_seq_t=[0 0.5/hpt_pwm_fs 1/hpt_pwm_fs]  rep_seq_y=[-1 1 -1]
  R_carrier_B2 : simulink/Sources/Repeating Sequence  rep_seq_t=[0 0.5/hpt_pwm_fs 1/hpt_pwm_fs]  rep_seq_y=[-1 1 -1]
  R_carrier_C1 : simulink/Sources/Repeating Sequence  rep_seq_t=[0 0.5/hpt_pwm_fs 1/hpt_pwm_fs]  rep_seq_y=[-1 1 -1]
  R_carrier_C2 : simulink/Sources/Repeating Sequence  rep_seq_t=[0 0.5/hpt_pwm_fs 1/hpt_pwm_fs]  rep_seq_y=[-1 1 -1]
  R_cmp_A1 : RelationalOperator  Operator=>  OutDataTypeStr=boolean  RndMeth=Simplest  InputSameDT=off
  R_cmp_A2 : RelationalOperator  Operator=>  OutDataTypeStr=boolean  RndMeth=Simplest  InputSameDT=off
  R_cmp_B1 : RelationalOperator  Operator=>  OutDataTypeStr=boolean  RndMeth=Simplest  InputSameDT=off
  R_cmp_B2 : RelationalOperator  Operator=>  OutDataTypeStr=boolean  RndMeth=Simplest  InputSameDT=off
  R_cmp_C1 : RelationalOperator  Operator=>  OutDataTypeStr=boolean  RndMeth=Simplest  InputSameDT=off
  R_cmp_C2 : RelationalOperator  Operator=>  OutDataTypeStr=boolean  RndMeth=Simplest  InputSameDT=off
  R_gate_mux_A : Mux
  R_gate_mux_B : Mux
  R_gate_mux_C : Mux
  R_not_A1 : Logic  Operator=NOT  AllPortsSameDT=off  OutDataTypeStr=boolean
  R_not_A2 : Logic  Operator=NOT  AllPortsSameDT=off  OutDataTypeStr=boolean
  R_not_B1 : Logic  Operator=NOT  AllPortsSameDT=off  OutDataTypeStr=boolean
  R_not_B2 : Logic  Operator=NOT  AllPortsSameDT=off  OutDataTypeStr=boolean
  R_not_C1 : Logic  Operator=NOT  AllPortsSameDT=off  OutDataTypeStr=boolean
  R_not_C2 : Logic  Operator=NOT  AllPortsSameDT=off  OutDataTypeStr=boolean
  m_ref_demux : Demux  Outputs=6
  HBC_A_1 : PMIOPort  Side=Left
  HBC_A_2 : PMIOPort  Port=2  Side=Left
  HBC_B_1 : PMIOPort  Port=3  Side=Left
  HBC_B_2 : PMIOPort  Port=4  Side=Left
  HBC_C_1 : PMIOPort  Port=5  Side=Left
  HBC_C_2 : PMIOPort  Port=6  Side=Left
  DC_pos : PMIOPort  Port=7  Side=Right
  DC_neg : PMIOPort  Port=8  Side=Right
  wires:
  m_ref6/1 -> m_ref_demux/1
  m_ref_demux/1 -> R_cmp_A1/1
  R_carrier_A1/1 -> R_cmp_A1/2
  R_cmp_A1/1 -> R_gate_mux_A/1, R_not_A1/1
  R_not_A1/1 -> R_gate_mux_A/2
  m_ref_demux/2 -> R_cmp_A2/1
  R_carrier_A2/1 -> R_cmp_A2/2
  R_cmp_A2/1 -> R_gate_mux_A/3, R_not_A2/1
  R_not_A2/1 -> R_gate_mux_A/4
  R_gate_mux_A/1 -> R_UB_A/1
  m_ref_demux/3 -> R_cmp_B1/1
  R_carrier_B1/1 -> R_cmp_B1/2
  R_cmp_B1/1 -> R_gate_mux_B/1, R_not_B1/1
  R_not_B1/1 -> R_gate_mux_B/2
  m_ref_demux/4 -> R_cmp_B2/1
  R_carrier_B2/1 -> R_cmp_B2/2
  R_cmp_B2/1 -> R_gate_mux_B/3, R_not_B2/1
  R_not_B2/1 -> R_gate_mux_B/4
  R_gate_mux_B/1 -> R_UB_B/1
  m_ref_demux/5 -> R_cmp_C1/1
  R_carrier_C1/1 -> R_cmp_C1/2
  R_cmp_C1/1 -> R_gate_mux_C/1, R_not_C1/1
  R_not_C1/1 -> R_gate_mux_C/2
  m_ref_demux/6 -> R_cmp_C2/1
  R_carrier_C2/1 -> R_cmp_C2/2
  R_cmp_C2/1 -> R_gate_mux_C/3, R_not_C2/1
  R_not_C2/1 -> R_gate_mux_C/4
  R_gate_mux_C/1 -> R_UB_C/1
  connections:
  HBC_A_1/RConn1 -- R_UB_A/LConn1
  HBC_A_2/RConn1 -- R_UB_A/LConn2
  HBC_B_1/RConn1 -- R_UB_B/LConn1
  HBC_B_2/RConn1 -- R_UB_B/LConn2
  HBC_C_1/RConn1 -- R_UB_C/LConn1
  HBC_C_2/RConn1 -- R_UB_C/LConn2
  R_UB_A/RConn1 -- DC_pos/RConn1 -- R_UB_B/RConn1 -- R_UB_C/RConn1
  R_UB_A/RConn2 -- R_UB_B/RConn2 -- DC_neg/RConn1 -- R_UB_C/RConn2

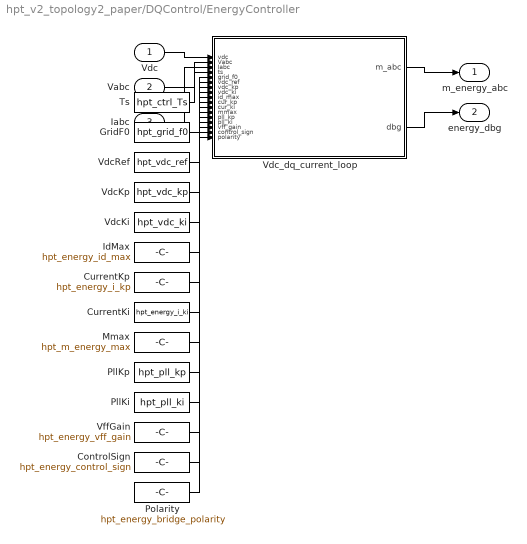
== system hpt_v2_topology2_paper/DQControl/EnergyController ==
  Vdc : Inport
  Vabc : Inport  Port=2
  Iabc : Inport  Port=3
  ControlSign : Constant  Value=hpt_energy_control_sign
  CurrentKi : Constant  Value=hpt_energy_i_ki
  CurrentKp : Constant  Value=hpt_energy_i_kp
  GridF0 : Constant  Value=hpt_grid_f0
  IdMax : Constant  Value=hpt_energy_id_max
  Mmax : Constant  Value=hpt_m_energy_max
  PllKi : Constant  Value=hpt_pll_ki
  PllKp : Constant  Value=hpt_pll_kp
  Polarity : Constant  Value=hpt_energy_bridge_polarity
  Ts : Constant  Value=hpt_ctrl_Ts
  VdcKi : Constant  Value=hpt_vdc_ki
  VdcKp : Constant  Value=hpt_vdc_kp
  VdcRef : Constant  Value=hpt_vdc_ref
  Vdc_dq_current_loop : MATLAB Function  TreatAsAtomicUnit=on
  VffGain : Constant  Value=hpt_energy_vff_gain
  m_energy_abc : Outport
  energy_dbg : Outport  Port=2
  wires:
  Ts/1 -> Vdc_dq_current_loop/4(ts)
  GridF0/1 -> Vdc_dq_current_loop/5(grid_f0)
  VdcRef/1 -> Vdc_dq_current_loop/6(vdc_ref)
  VdcKp/1 -> Vdc_dq_current_loop/7(vdc_kp)
  VdcKi/1 -> Vdc_dq_current_loop/8(vdc_ki)
  IdMax/1 -> Vdc_dq_current_loop/9(id_max)
  CurrentKp/1 -> Vdc_dq_current_loop/10(cur_kp)
  CurrentKi/1 -> Vdc_dq_current_loop/11(cur_ki)
  Mmax/1 -> Vdc_dq_current_loop/12(mmax)
  PllKp/1 -> Vdc_dq_current_loop/13(pll_kp)
  PllKi/1 -> Vdc_dq_current_loop/14(pll_ki)
  VffGain/1 -> Vdc_dq_current_loop/15(vff_gain)
  ControlSign/1 -> Vdc_dq_current_loop/16(control_sign)
  Polarity/1 -> Vdc_dq_current_loop/17(polarity)
  Vdc/1 -> Vdc_dq_current_loop/1(vdc)
  Vabc/1 -> Vdc_dq_current_loop/2(Vabc)
  Iabc/1 -> Vdc_dq_current_loop/3(Iabc)
  Vdc_dq_current_loop/1(m_abc) -> m_energy_abc/1
  Vdc_dq_current_loop/2(dbg) -> energy_dbg/1

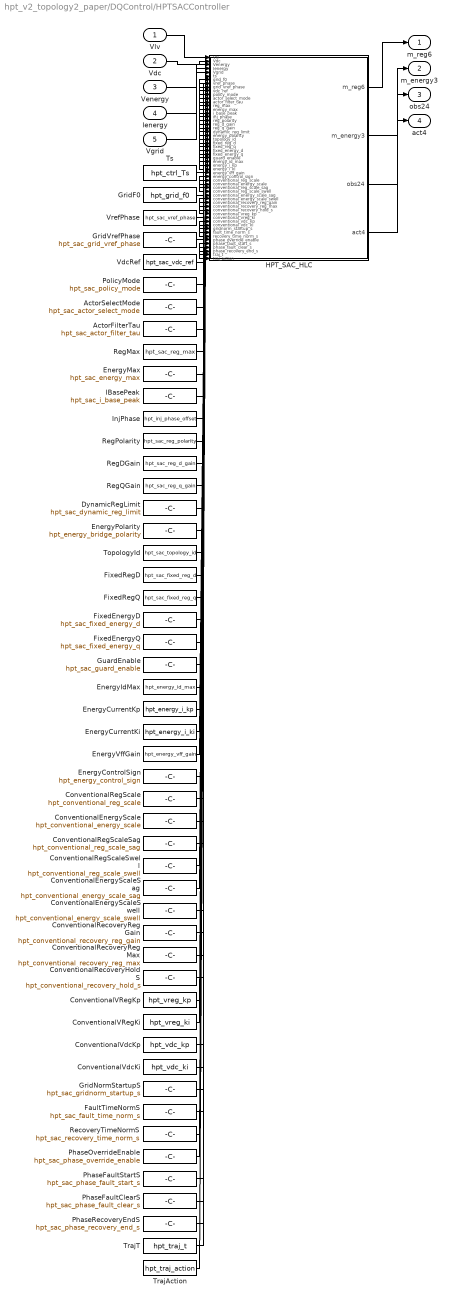
== system hpt_v2_topology2_paper/DQControl/HPTSACController ==
  Vlv : Inport
  Vdc : Inport  Port=2
  Venergy : Inport  Port=3
  Ienergy : Inport  Port=4
  Vgrid : Inport  Port=5
  ActorFilterTau : Constant  Value=hpt_sac_actor_filter_tau
  ActorSelectMode : Constant  Value=hpt_sac_actor_select_mode
  ConventionalEnergyScale : Constant  Value=hpt_conventional_energy_scale
  ConventionalEnergyScaleSag : Constant  Value=hpt_conventional_energy_scale_sag
  ConventionalEnergyScaleSwell : Constant  Value=hpt_conventional_energy_scale_swell
  ConventionalRecoveryHoldS : Constant  Value=hpt_conventional_recovery_hold_s
  ConventionalRecoveryRegGain : Constant  Value=hpt_conventional_recovery_reg_gain
  ConventionalRecoveryRegMax : Constant  Value=hpt_conventional_recovery_reg_max
  ConventionalRegScale : Constant  Value=hpt_conventional_reg_scale
  ConventionalRegScaleSag : Constant  Value=hpt_conventional_reg_scale_sag
  ConventionalRegScaleSwell : Constant  Value=hpt_conventional_reg_scale_swell
  ConventionalVRegKi : Constant  Value=hpt_vreg_ki
  ConventionalVRegKp : Constant  Value=hpt_vreg_kp
  ConventionalVdcKi : Constant  Value=hpt_vdc_ki
  ConventionalVdcKp : Constant  Value=hpt_vdc_kp
  DynamicRegLimit : Constant  Value=hpt_sac_dynamic_reg_limit
  EnergyControlSign : Constant  Value=hpt_energy_control_sign
  EnergyCurrentKi : Constant  Value=hpt_energy_i_ki
  EnergyCurrentKp : Constant  Value=hpt_energy_i_kp
  EnergyIdMax : Constant  Value=hpt_energy_id_max
  EnergyMax : Constant  Value=hpt_sac_energy_max
  EnergyPolarity : Constant  Value=hpt_energy_bridge_polarity
  EnergyVffGain : Constant  Value=hpt_energy_vff_gain
  FaultTimeNormS : Constant  Value=hpt_sac_fault_time_norm_s
  FixedEnergyD : Constant  Value=hpt_sac_fixed_energy_d
  FixedEnergyQ : Constant  Value=hpt_sac_fixed_energy_q
  FixedRegD : Constant  Value=hpt_sac_fixed_reg_d
  FixedRegQ : Constant  Value=hpt_sac_fixed_reg_q
  GridF0 : Constant  Value=hpt_grid_f0
  GridNormStartupS : Constant  Value=hpt_sac_gridnorm_startup_s
  GridVrefPhase : Constant  Value=hpt_sac_grid_vref_phase
  GuardEnable : Constant  Value=hpt_sac_guard_enable
  HPT_SAC_HLC : MATLAB Function  TreatAsAtomicUnit=on
  IBasePeak : Constant  Value=hpt_sac_i_base_peak
  InjPhase : Constant  Value=hpt_inj_phase_offset
  PhaseFaultClearS : Constant  Value=hpt_sac_phase_fault_clear_s
  PhaseFaultStartS : Constant  Value=hpt_sac_phase_fault_start_s
  PhaseOverrideEnable : Constant  Value=hpt_sac_phase_override_enable
  PhaseRecoveryEndS : Constant  Value=hpt_sac_phase_recovery_end_s
  PolicyMode : Constant  Value=hpt_sac_policy_mode
  RecoveryTimeNormS : Constant  Value=hpt_sac_recovery_time_norm_s
  RegDGain : Constant  Value=hpt_sac_reg_d_gain
  RegMax : Constant  Value=hpt_sac_reg_max
  RegPolarity : Constant  Value=hpt_sac_reg_polarity
  RegQGain : Constant  Value=hpt_sac_reg_q_gain
  TopologyId : Constant  Value=hpt_sac_topology_id
  TrajAction : Constant  Value=hpt_traj_action
  TrajT : Constant  Value=hpt_traj_t
  Ts : Constant  Value=hpt_ctrl_Ts
  VdcRef : Constant  Value=hpt_sac_vdc_ref
  VrefPhase : Constant  Value=hpt_sac_vref_phase
  m_reg6 : Outport
  m_energy3 : Outport  Port=2
  obs24 : Outport  Port=3
  act4 : Outport  Port=4
  wires:
  Ts/1 -> HPT_SAC_HLC/6(ts)
  GridF0/1 -> HPT_SAC_HLC/7(grid_f0)
  VrefPhase/1 -> HPT_SAC_HLC/8(vref_phase)
  GridVrefPhase/1 -> HPT_SAC_HLC/9(grid_vref_phase)
  VdcRef/1 -> HPT_SAC_HLC/10(vdc_ref)
  PolicyMode/1 -> HPT_SAC_HLC/11(policy_mode)
  ActorSelectMode/1 -> HPT_SAC_HLC/12(actor_select_mode)
  ActorFilterTau/1 -> HPT_SAC_HLC/13(actor_filter_tau)
  RegMax/1 -> HPT_SAC_HLC/14(reg_max)
  EnergyMax/1 -> HPT_SAC_HLC/15(energy_max)
  IBasePeak/1 -> HPT_SAC_HLC/16(i_base_peak)
  InjPhase/1 -> HPT_SAC_HLC/17(inj_phase)
  RegPolarity/1 -> HPT_SAC_HLC/18(reg_polarity)
  RegDGain/1 -> HPT_SAC_HLC/19(reg_d_gain)
  RegQGain/1 -> HPT_SAC_HLC/20(reg_q_gain)
  DynamicRegLimit/1 -> HPT_SAC_HLC/21(dynamic_reg_limit)
  EnergyPolarity/1 -> HPT_SAC_HLC/22(energy_polarity)
  TopologyId/1 -> HPT_SAC_HLC/23(topology_id)
  FixedRegD/1 -> HPT_SAC_HLC/24(fixed_reg_d)
  FixedRegQ/1 -> HPT_SAC_HLC/25(fixed_reg_q)
  FixedEnergyD/1 -> HPT_SAC_HLC/26(fixed_energy_d)
  FixedEnergyQ/1 -> HPT_SAC_HLC/27(fixed_energy_q)
  GuardEnable/1 -> HPT_SAC_HLC/28(guard_enable)
  EnergyIdMax/1 -> HPT_SAC_HLC/29(energy_id_max)
  EnergyCurrentKp/1 -> HPT_SAC_HLC/30(energy_i_kp)
  EnergyCurrentKi/1 -> HPT_SAC_HLC/31(energy_i_ki)
  EnergyVffGain/1 -> HPT_SAC_HLC/32(energy_vff_gain)
  EnergyControlSign/1 -> HPT_SAC_HLC/33(energy_control_sign)
  ConventionalRegScale/1 -> HPT_SAC_HLC/34(conventional_reg_scale)
  ConventionalEnergyScale/1 -> HPT_SAC_HLC/35(conventional_energy_scale)
  ConventionalRegScaleSag/1 -> HPT_SAC_HLC/36(conventional_reg_scale_sag)
  ConventionalRegScaleSwell/1 -> HPT_SAC_HLC/37(conventional_reg_scale_swell)
  ConventionalEnergyScaleSag/1 -> HPT_SAC_HLC/38(conventional_energy_scale_sag)
  ConventionalEnergyScaleSwell/1 -> HPT_SAC_HLC/39(conventional_energy_scale_swell)
  ConventionalRecoveryRegGain/1 -> HPT_SAC_HLC/40(conventional_recovery_reg_gain)
  ConventionalRecoveryRegMax/1 -> HPT_SAC_HLC/41(conventional_recovery_reg_max)
  ConventionalRecoveryHoldS/1 -> HPT_SAC_HLC/42(conventional_recovery_hold_s)
  ConventionalVRegKp/1 -> HPT_SAC_HLC/43(conventional_vreg_kp)
  ConventionalVRegKi/1 -> HPT_SAC_HLC/44(conventional_vreg_ki)
  ConventionalVdcKp/1 -> HPT_SAC_HLC/45(conventional_vdc_kp)
  ConventionalVdcKi/1 -> HPT_SAC_HLC/46(conventional_vdc_ki)
  GridNormStartupS/1 -> HPT_SAC_HLC/47(gridnorm_startup_s)
  FaultTimeNormS/1 -> HPT_SAC_HLC/48(fault_time_norm_s)
  RecoveryTimeNormS/1 -> HPT_SAC_HLC/49(recovery_time_norm_s)
  PhaseOverrideEnable/1 -> HPT_SAC_HLC/50(phase_override_enable)
  PhaseFaultStartS/1 -> HPT_SAC_HLC/51(phase_fault_start_s)
  PhaseFaultClearS/1 -> HPT_SAC_HLC/52(phase_fault_clear_s)
  PhaseRecoveryEndS/1 -> HPT_SAC_HLC/53(phase_recovery_end_s)
  TrajT/1 -> HPT_SAC_HLC/54(traj_t)
  TrajAction/1 -> HPT_SAC_HLC/55(traj_action)
  Vlv/1 -> HPT_SAC_HLC/1(Vlv)
  Vdc/1 -> HPT_SAC_HLC/2(Vdc)
  Venergy/1 -> HPT_SAC_HLC/3(Venergy)
  Ienergy/1 -> HPT_SAC_HLC/4(Ienergy)
  Vgrid/1 -> HPT_SAC_HLC/5(Vgrid)
  HPT_SAC_HLC/1(m_reg6) -> m_reg6/1
  HPT_SAC_HLC/2(m_energy3) -> m_energy3/1
  HPT_SAC_HLC/3(obs24) -> obs24/1
  HPT_SAC_HLC/4(act4) -> act4/1

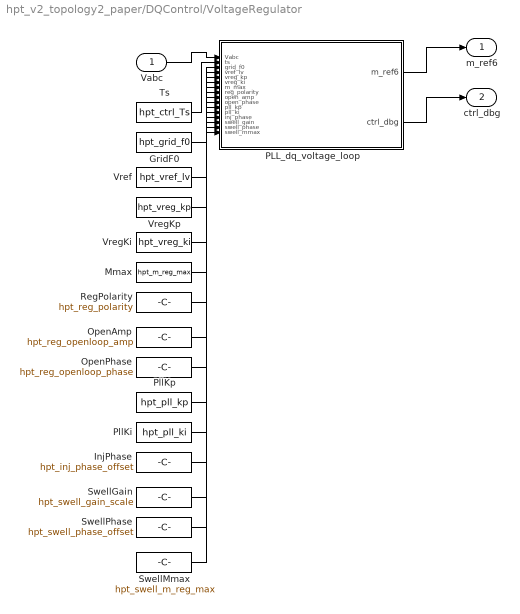
== system hpt_v2_topology2_paper/DQControl/VoltageRegulator ==
  Vabc : Inport
  GridF0 : Constant  Value=hpt_grid_f0
  InjPhase : Constant  Value=hpt_inj_phase_offset
  Mmax : Constant  Value=hpt_m_reg_max
  OpenAmp : Constant  Value=hpt_reg_openloop_amp
  OpenPhase : Constant  Value=hpt_reg_openloop_phase
  PLL_dq_voltage_loop : MATLAB Function  TreatAsAtomicUnit=on
  PllKi : Constant  Value=hpt_pll_ki
  PllKp : Constant  Value=hpt_pll_kp
  RegPolarity : Constant  Value=hpt_reg_polarity
  SwellGain : Constant  Value=hpt_swell_gain_scale
  SwellMmax : Constant  Value=hpt_swell_m_reg_max
  SwellPhase : Constant  Value=hpt_swell_phase_offset
  Ts : Constant  Value=hpt_ctrl_Ts
  Vref : Constant  Value=hpt_vref_lv
  VregKi : Constant  Value=hpt_vreg_ki
  VregKp : Constant  Value=hpt_vreg_kp
  m_ref6 : Outport
  ctrl_dbg : Outport  Port=2
  wires:
  Ts/1 -> PLL_dq_voltage_loop/2(ts)
  GridF0/1 -> PLL_dq_voltage_loop/3(grid_f0)
  Vref/1 -> PLL_dq_voltage_loop/4(vref_lv)
  VregKp/1 -> PLL_dq_voltage_loop/5(vreg_kp)
  VregKi/1 -> PLL_dq_voltage_loop/6(vreg_ki)
  Mmax/1 -> PLL_dq_voltage_loop/7(m_max)
  RegPolarity/1 -> PLL_dq_voltage_loop/8(reg_polarity)
  OpenAmp/1 -> PLL_dq_voltage_loop/9(open_amp)
  OpenPhase/1 -> PLL_dq_voltage_loop/10(open_phase)
  PllKp/1 -> PLL_dq_voltage_loop/11(pll_kp)
  PllKi/1 -> PLL_dq_voltage_loop/12(pll_ki)
  InjPhase/1 -> PLL_dq_voltage_loop/13(inj_phase)
  SwellGain/1 -> PLL_dq_voltage_loop/14(swell_gain)
  SwellPhase/1 -> PLL_dq_voltage_loop/15(swell_phase)
  SwellMmax/1 -> PLL_dq_voltage_loop/16(swell_mmax)
  Vabc/1 -> PLL_dq_voltage_loop/1(Vabc)
  PLL_dq_voltage_loop/1(m_ref6) -> m_ref6/1
  PLL_dq_voltage_loop/2(ctrl_dbg) -> ctrl_dbg/1
